simulink model "zrf_volt_4ant"  (R2019a)
settings: Solver=VariableStepAuto  StartTime=0.0  StopTime=10.0  RelTol=1e-3
libraries: xbsIndex_r4 x6321, casper_library_misc x95, xps_library x10, casper_library_delays x1
(part 1 of 63)
settings Model: Creator=jackh  LastModifiedBy=jackh

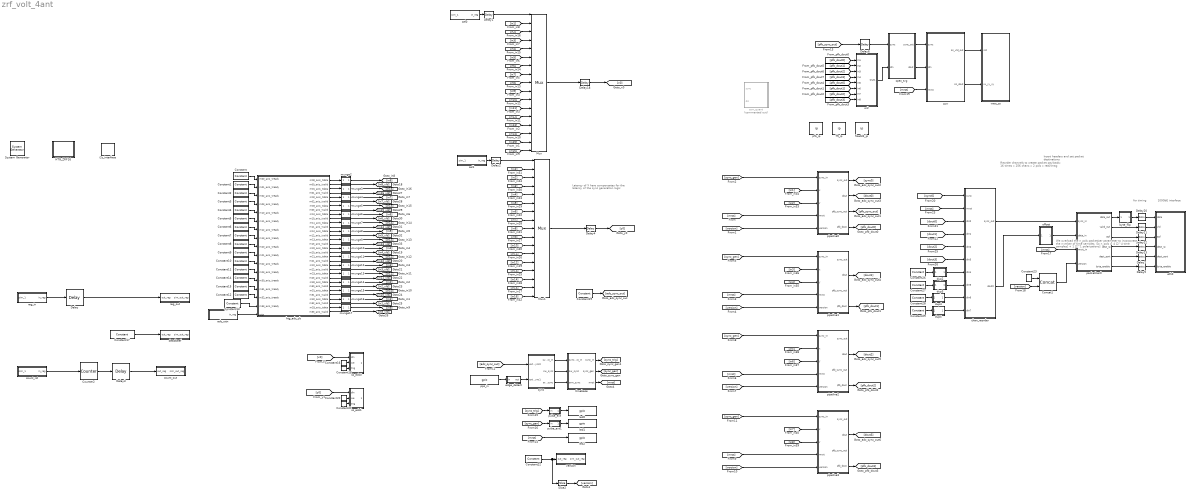
== system zrf_volt_4ant ==
  note: Latency of 5 here compensates
      | for the latency of the sync generation logic
  note: 100GbE interface
  note: for timing
  note: Insert headers and
      | set packet destinations
  note: We overload the n_pols packetizer
      | parameter to incorporate the number of time samples.
      | So n_pols = 4 [2^4 time samples] + 1 [2^1 polarizations]
  note: Reorder channels to
      | create packet payloads:
      | 16 times x 256 chans x 2 pols x real/imag
  " System Generator" : xbsIndex_r4/ System Generator  Tag=genX  xilinxfamily=zynquplusRFSOC  part=xczu49dr  speed=-2-e  package=ffvf1760  synthesis_tool=XST  clock_wrapper=Clock Enables  directory=/home/jackh/src/ata_rfsoc/zrf_volt_4ant/sysgen  proj_type=Vivado  Synth_file=Vivado Synthesis Defaults  Impl_file=Vivado Implementation Defaults  testbench=off  simulink_period=1  sysclk_period=3.9062  dcm_input_clock_period=10  incr_netlist=off  trim_vbits=Everywhere in SubSystem  dbl_ovrd=According to Block Masks  core_generation=According to Block Masks  run_coregen=off  deprecated_control=off  eval_field=0  block_type=sysgen
  Concat1 : xbsIndex_r4/Concat  num_inputs=2  dbl_ovrd=off  block_type=concat
  Constant{,1..15} (16 alike) : xbsIndex_r4/Constant  const=1  gui_display_data_type=Boolean  arith_type=Boolean  n_bits=1  bin_pt=0  preci_type=Single  exp_width=8  frac_width=24  explicit_period=on  period=1  equ=P=C  opselect=C  inp2=PCIN>>17  opr=+  inp1=P  carry=CIN  dbl_ovrd=off  block_type=constant
  Constant{16,18..21} (5 alike) : xbsIndex_r4/Constant  const=0  gui_display_data_type=Boolean  arith_type=Boolean  n_bits=16  bin_pt=14  preci_type=Single  exp_width=8  frac_width=24  explicit_period=on  period=1  equ=P=C  opselect=C  inp2=PCIN>>17  opr=+  inp1=P  carry=CIN  dbl_ovrd=off  block_type=constant
  Constant17 : xbsIndex_r4/Constant  const=hex2dec('deadbeef')  gui_display_data_type=Fixed-point  arith_type=Unsigned  n_bits=32  bin_pt=0  preci_type=Single  exp_width=8  frac_width=24  explicit_period=on  period=1  equ=P=C  opselect=C  inp2=PCIN>>17  opr=+  inp1=P  carry=CIN  dbl_ovrd=off  block_type=constant
  Constant22 : xbsIndex_r4/Constant  const=2  gui_display_data_type=Fixed-point  arith_type=Unsigned  n_bits=7  bin_pt=0  preci_type=Single  exp_width=8  frac_width=24  explicit_period=on  period=1  equ=P=C  opselect=C  inp2=PCIN>>17  opr=+  inp1=P  carry=CIN  dbl_ovrd=off  block_type=constant
  Constant23 : xbsIndex_r4/Constant  const=0  gui_display_data_type=Fixed-point  arith_type=Unsigned  n_bits=1  bin_pt=0  preci_type=Single  exp_width=8  frac_width=24  explicit_period=on  period=1  equ=P=C  opselect=C  inp2=PCIN>>17  opr=+  inp1=P  carry=CIN  dbl_ovrd=off  block_type=constant
  Constant26 : xbsIndex_r4/Constant  const=4  gui_display_data_type=Fixed-point  arith_type=Unsigned  n_bits=8  bin_pt=0  preci_type=Single  exp_width=8  frac_width=24  explicit_period=on  period=1  equ=P=C  opselect=C  inp2=PCIN>>17  opr=+  inp1=P  carry=CIN  dbl_ovrd=off  block_type=constant
  Constant27 : xbsIndex_r4/Constant  const=5  gui_display_data_type=Fixed-point  arith_type=Unsigned  n_bits=8  bin_pt=0  preci_type=Single  exp_width=8  frac_width=24  explicit_period=on  period=1  equ=P=C  opselect=C  inp2=PCIN>>17  opr=+  inp1=P  carry=CIN  dbl_ovrd=off  block_type=constant
  Constant28 : xbsIndex_r4/Constant  const=6  gui_display_data_type=Fixed-point  arith_type=Unsigned  n_bits=8  bin_pt=0  preci_type=Single  exp_width=8  frac_width=24  explicit_period=on  period=1  equ=P=C  opselect=C  inp2=PCIN>>17  opr=+  inp1=P  carry=CIN  dbl_ovrd=off  block_type=constant
  Constant29 : xbsIndex_r4/Constant  const=7  gui_display_data_type=Fixed-point  arith_type=Unsigned  n_bits=8  bin_pt=0  preci_type=Single  exp_width=8  frac_width=24  explicit_period=on  period=1  equ=P=C  opselect=C  inp2=PCIN>>17  opr=+  inp1=P  carry=CIN  dbl_ovrd=off  block_type=constant
  Counter2 : xbsIndex_r4/Counter  cnt_type=Free Running  cnt_to=Inf  operation=Up  start_count=0  cnt_by_val=1  arith_type=Unsigned  n_bits=32  bin_pt=0  load_pin=off  rst=on  en=off  explicit_period=on  period=1  use_behavioral_HDL=off  implementation=DSP48  dbl_ovrd=off  block_type=counter
  Delay{,1..3,5,7,20..23} (10 alike) : xbsIndex_r4/Delay  rst=off  infoeditControl=Selection of Reset will increase slice count due to use of real FFs and instead of SRLs  en=off  latency=1  reg_retiming=off  dbl_ovrd=off  block_type=delay
      Delay1 settings: block_version=11.4
      Delay2 settings: block_version=11.4
  Delay18 : xbsIndex_r4/Delay  rst=off  infoeditControl=Selection of Reset will increase slice count due to use of real FFs and instead of SRLs  en=off  latency=5  reg_retiming=off  dbl_ovrd=off  block_type=delay
      settings: block_version=11.4
  Delay4 : xbsIndex_r4/Delay  rst=off  infoeditControl=Selection of Reset will increase slice count due to use of real FFs and instead of SRLs  en=off  latency=5  reg_retiming=off  dbl_ovrd=off  block_type=delay
      settings: block_version=11.4
  Delay6 : xbsIndex_r4/Delay  rst=off  infoeditControl=Selection of Reset will increase slice count due to use of real FFs and instead of SRLs  en=off  latency=2  reg_retiming=off  dbl_ovrd=off  block_type=delay
  HTG_ZRF16 : Subsystem  Tag=xps:xsg  mask(xsg core config){hw_sys=htg_zrf16:xczu49dr, clk_src=adc_clk, clk_rate=256, sample_period=1, synthesis_tool=XST}
      mask prompts: hw_sys "Hardware Platform"; clk_src "User IP Clock source"; clk_rate "User IP Clock Rate (MHz)"; sample_period "Sample Period"; synthesis_tool "Synthesis Tool:"
      mask help:
      | The XSG Core Config block is used to configure the System Generator design
      | for the casper_xps toolflow. Settings here are used to configure the
      | Xilinx System Generator block parameters automatically, and control toolflow
      | script  execution. It needs to be at the top level of all designs being compiled
      | with the casper_xps toolflow.
      mask init:
      | xps_xsg_htg_zrf16_conf_mask;
      mask Help: eval('xlWeb([getenv(''MLIB_ROOT''), ''\doc\html\sys_xsg_core_config\sys_xsg_core_config.html''])')
      mask TypeOptions hw_sys: htg_zrf16:xczu29dr | htg_zrf16:xczu49dr
      mask TypeOptions clk_src: sys_clk | adc_clk | arb_clk
      mask TypeOptions synthesis_tool: Leonardo Spectrum | Synplify | Synplify Pro | XST
      mask Display: fprintf(['ZRF16']);
  Mux : xbsIndex_r4/Mux  inputs=16  en=off  latency=2  precision=Full  arith_type=Unsigned  n_bits=16  bin_pt=14  quantization=Truncate  overflow=Wrap  dbl_ovrd=off  block_type=mux
  Mux1 : xbsIndex_r4/Mux  inputs=16  en=off  latency=2  precision=Full  arith_type=Unsigned  n_bits=16  bin_pt=14  quantization=Truncate  overflow=Wrap  dbl_ovrd=off  block_type=mux
  Slice2 : xbsIndex_r4/Slice  nbits=7  boolean_output=off  mode=Lower Bit Location + Width  bit1=0  base1=MSB of Input  bit0=0  base0=LSB of Input  dbl_ovrd=off  block_type=slice
  adc_rstn : Subsystem  Tag=xps:sw_reg  AncestorBlock=xps_library/Memory/software_register  mask(swreg){io_dir=From Processor, io_delay=0, init_val=0, sample_period=1, names=reg, bitwidths=1, bin_pts=0, arith_types=2, sim_port=off, show_format=on}
      mask prompts: io_dir "I/O direction"; io_delay "I/O delay"; init_val "Initial Value"; sample_period "Sample period"; names "Bitfield names [msb...lsb]"; bitwidths "Bitfield widths"; bin_pts "Bitfield binary pts"; arith_types "Bitfield types, ufix=0, fix=1, bool=2"; sim_port "Provide sim input/output?"; show_format "Print format string?"
      mask help: A 32-bit software-accessible register. Can be divided into bitfields of varying widths and types using the fields in the block mask.
      mask init:
      | swreg_init(gcb)
      settings: AttributesFormatString=1input:b = 1 bits
      mask TypeOptions io_dir: To Processor | From Processor
      mask Callback io_dir:
      | mask_enables = get_param(gcb, 'MaskEnables');
      | mask_names = get_param(gcb, 'MaskNames');
      | if strcmp(get_param(gcb, 'io_dir'), 'To Processor'),
      |     mask_enables{ismember(mask_names, 'sample_period')} = 'off';
      | else
      |     mask_enables{ismember(mask_names, 'sample_period')} = 'on';
      | end
      | set_param(gcb, 'MaskEnables', mask_enables);
      mask DialogControl ParameterTabVar0 Prompt: Setup
  byte_flip : Subsystem  AncestorBlock=casper_library_flow_control/munge  mask(munge){divisions=64, div_size=8*ones(1,64), order=[63:-1:0], arith_type_out=Unsigned, bin_pt_out=0}
      mask prompts: divisions "Number of divisions"; div_size "Division size (bits)"; order "Division packing order"; arith_type_out "Output arithmetic type"; bin_pt_out "Output binary point"
      mask help: Splits an input bus into the specified number of divisions and then recombines them in the order specified (most significant division = 0,least = number divisions-1)
      mask init:
      | munge_init(gcb, ...
      |     'divisions', divisions, ...
      |     'div_size', div_size, ...
      |     'order', order, ...
      |     'arith_type_out', arith_type_out, ...
      |     'bin_pt_out', bin_pt_out);
      settings: AttributesFormatString=|
      | split:[8 8 8 8 8 8 8 8 8 8 8 8 8 8 8 8 8 8 8 8 8 8 8 8 8 8 8 8 8 8 8 8 8 8 8 8 8 8 8 8 8 8 8 8 8 8 8 8 8 8 8 8 8 8 8 8 8 8 8 8 8 8 8 8]
      | join:[63 62 61 60 59 58 57 56 55 54 53 52 51 50 49 48 47 46 45 44 43 42 41 40 39 38 37 36 35 34 33 32 31 30 29 28 27 26 25 24 23 22 21 20 19 18 17 16 15 14 13 12 11 10 9 8 7 6 5 4 3 2 1 0]
      | Unsigned [512,0]
      mask TypeOptions arith_type_out: Unsigned | Signed  (2's comp) | Floating-point
  chan_reorder : Subsystem
  corr : Subsystem  mask{n_chan_bits=12}
      mask prompts: n_chan_bits "Number of channels? (2^?)"
  corr_quant : Subsystem  Commented=on  mask{n_chan_bits=12}
      mask prompts: n_chan_bits "Number of channels? (2^?)"
  count_out : Subsystem  Tag=xps:sw_reg  AncestorBlock=xps_library/Memory/software_register  mask(swreg){io_dir=To Processor, io_delay=0, init_val=0, sample_period=1, names=reg, bitwidths=32, bin_pts=0, arith_types=0, sim_port=on, show_format=on}
      mask prompts: io_dir "I/O direction"; io_delay "I/O delay"; init_val "Initial Value"; sample_period "Sample period"; names "Bitfield names [msb...lsb]"; bitwidths "Bitfield widths"; bin_pts "Bitfield binary pts"; arith_types "Bitfield types, ufix=0, fix=1, bool=2"; sim_port "Provide sim input/output?"; show_format "Print format string?"
      mask help: A 32-bit software-accessible register. Can be divided into bitfields of varying widths and types using the fields in the block mask.
      mask init:
      | swreg_init(gcb)
      settings: AttributesFormatString=1output:uf32.0 = 32 bits
      mask TypeOptions io_dir: To Processor | From Processor
      mask Callback io_dir:
      | mask_enables = get_param(gcb, 'MaskEnables');
      | mask_names = get_param(gcb, 'MaskNames');
      | if strcmp(get_param(gcb, 'io_dir'), 'To Processor'),
      |     mask_enables{ismember(mask_names, 'sample_period')} = 'off';
      | else
      |     mask_enables{ismember(mask_names, 'sample_period')} = 'on';
      | end
      | set_param(gcb, 'MaskEnables', mask_enables);
      mask DialogControl ParameterTabVar0 Prompt: Setup
  count_rst : Subsystem  Tag=xps:sw_reg  AncestorBlock=xps_library/Memory/software_register  mask(swreg){io_dir=From Processor, io_delay=0, init_val=0, sample_period=1, names=reg, bitwidths=1, bin_pts=0, arith_types=2, sim_port=on, show_format=on}
      mask prompts: io_dir "I/O direction"; io_delay "I/O delay"; init_val "Initial Value"; sample_period "Sample period"; names "Bitfield names [msb...lsb]"; bitwidths "Bitfield widths"; bin_pts "Bitfield binary pts"; arith_types "Bitfield types, ufix=0, fix=1, bool=2"; sim_port "Provide sim input/output?"; show_format "Print format string?"
      mask help: A 32-bit software-accessible register. Can be divided into bitfields of varying widths and types using the fields in the block mask.
      mask init:
      | swreg_init(gcb)
      settings: AttributesFormatString=1input:b = 1 bits
      mask TypeOptions io_dir: To Processor | From Processor
      mask Callback io_dir:
      | mask_enables = get_param(gcb, 'MaskEnables');
      | mask_names = get_param(gcb, 'MaskNames');
      | if strcmp(get_param(gcb, 'io_dir'), 'To Processor'),
      |     mask_enables{ismember(mask_names, 'sample_period')} = 'off';
      | else
      |     mask_enables{ismember(mask_names, 'sample_period')} = 'on';
      | end
      | set_param(gcb, 'MaskEnables', mask_enables);
      mask DialogControl ParameterTabVar0 Prompt: Setup
  deadbeef : Subsystem  Tag=xps:sw_reg  AncestorBlock=xps_library/Memory/software_register  mask(swreg){io_dir=To Processor, io_delay=0, init_val=0, sample_period=1, names=reg, bitwidths=32, bin_pts=0, arith_types=0, sim_port=on, show_format=on}
      mask prompts: io_dir "I/O direction"; io_delay "I/O delay"; init_val "Initial Value"; sample_period "Sample period"; names "Bitfield names [msb...lsb]"; bitwidths "Bitfield widths"; bin_pts "Bitfield binary pts"; arith_types "Bitfield types, ufix=0, fix=1, bool=2"; sim_port "Provide sim input/output?"; show_format "Print format string?"
      mask help: A 32-bit software-accessible register. Can be divided into bitfields of varying widths and types using the fields in the block mask.
      mask init:
      | swreg_init(gcb)
      settings: AttributesFormatString=1output:uf32.0 = 32 bits
      mask TypeOptions io_dir: To Processor | From Processor
      mask Callback io_dir:
      | mask_enables = get_param(gcb, 'MaskEnables');
      | mask_names = get_param(gcb, 'MaskNames');
      | if strcmp(get_param(gcb, 'io_dir'), 'To Processor'),
      |     mask_enables{ismember(mask_names, 'sample_period')} = 'off';
      | else
      |     mask_enables{ismember(mask_names, 'sample_period')} = 'on';
      | end
      | set_param(gcb, 'MaskEnables', mask_enables);
      mask DialogControl ParameterTabVar0 Prompt: Setup
  dup2 : Subsystem
  dup3 : Subsystem
  dup4 : Subsystem
  dup5 : Subsystem
  edge_detect : Subsystem  AncestorBlock=casper_library_misc/edge_detect  mask(edge_detect){edge=Rising, polarity=Active High, x_in=[0 0.08 0.08 0.16 0.16 0.24 0.24 0.32 0.32 0.4], y_in=[-1 -1  1  1  1  1  1  1  1  1], x_out=[0.6 0.68 0.68 0.76 0.76 0.84 0.84 0.92 0.92 1], y_out=[-1 -1  1  1 -1 -1 -1 -1 -1 -1]}
      mask prompts: edge "Edge Type"; polarity "Output Polarity"; x_in "Input X Positions"; y_in "Input Y Positions"; x_out "Output X Positions"; y_out "Output Y Positions"
      mask help: Output is active for one-cycle after each edge of the specified type (i.e. rising, falling or both).
      mask init:
      | edge_detect_init(gcb,...
      |     'edge',edge,...
      |     'polarity',polarity,...
      |     'x_in',x_in,...
      |     'x_out',x_out,...
      |     'y_in',y_in,...
      |     'y_out',y_out);
      | 
      | x_in_num=str2num(getfield(getfield(get_param(gcb,'UserData'),'parameters'),'x_in'));
      | x_out_num=str2num(getfield(getfield(get_param(gcb,'UserData'),'parameters'),'x_out'));
      | y_in_num=str2num(getfield(getfield(get_param(gcb,'UserData'),'parameters'),'y_in'));
      | y_out_num=str2num(getfield(getfield(get_param(gcb,'UserData'),'parameters'),'y_out'));
      settings: AttributesFormatString=|
      | rising edges
      | active high
      mask Help: Output is active for one-cycle after each edge of the specified type (i.e. rising, falling, or both).  Latency is zero.
      mask TypeOptions edge: Rising | Falling | Both
      mask TypeOptions polarity: Active High | Active Low
      mask Display:
      | plot(x_in_num,0.5+y_in_num*0.2);
      | plot(x_out_num,0.5+y_out_num*0.2);
  eth0 : Subsystem
  fft_ip : xps_library/Utilities/ip  Tag=xps:ip  lib_path=[fileparts(which(bdroot)) '/fft_4096c_2i_core']  ip_name='fft_4096c_2i_core'
      settings: SourceProductName=CASPER XPS Blockset
  float32_ip : xps_library/Utilities/ip  Tag=xps:ip  lib_path=[fileparts(which(bdroot)) '/int64_to_float32_latency6_core']  ip_name='int64_to_float32_latency6_core'
      settings: SourceProductName=CASPER XPS Blockset
  htg_adc_yb : Subsystem  Tag=xps:adc_htgzrf16  mask(htg_adc){tile_224_enable_pll=on, tile_224_sample_rate=4096, tile_224_clk_out=256.000, tile_224_ref_clk=512.000, tile_224_axi_stream_clk=0, tile_224_adc_0=on, tile_224_adc0_digital_output=I/Q, tile_224_adc0_dec_mode=2x, tile_224_adc0_sample_per_cycle=8, tile_224_adc0_req_axis_clk=0, tile_224_adc_1=on, tile_224_adc1_digital_output=I/Q, tile_224_adc1_dec_mode=2x, tile_224_adc1_sample_per_cycle=8, tile_224_adc1_req_axis_clk=0, tile_225_enable_pll=on, tile_225_sample_rate=4096, tile_225_clk_out=256.000, tile_225_ref_clk=512.000, tile_225_axi_stream_clk=0, tile_225_adc_0=on, tile_225_adc0_digital_output=I/Q, tile_225_adc0_dec_mode=2x, tile_225_adc0_sample_per_cycle=8, tile_225_adc0_req_axis_clk=0, tile_225_adc_1=on, tile_225_adc1_digital_output=I/Q, tile_225_adc1_dec_mode=2x, tile_225_adc1_sample_per_cycle=8, tile_225_adc1_req_axis_clk=0, tile_226_enable_pll=on, tile_226_sample_rate=4096, tile_226_clk_out=256.000, tile_226_ref_clk=512.000, tile_226_axi_stream_clk=0, tile_226_adc_0=on, tile_226_adc0_digital_output=I/Q, tile_226_adc0_dec_mode=2x, tile_226_adc0_sample_per_cycle=8, tile_226_adc0_req_axis_clk=0, tile_226_adc_1=on, tile_226_adc1_digital_output=I/Q, tile_226_adc1_dec_mode=2x, tile_226_adc1_sample_per_cycle=8, tile_226_adc1_req_axis_clk=0, tile_227_enable_pll=on, tile_227_sample_rate=4096, tile_227_clk_out=256.000, tile_227_ref_clk=512.000, tile_227_axi_stream_clk=0, tile_227_adc_0=on, tile_227_adc0_digital_output=I/Q, tile_227_adc0_dec_mode=2x, tile_227_adc0_sample_per_cycle=8, tile_227_adc0_req_axis_clk=0, tile_227_adc_1=on, tile_227_adc1_digital_output=I/Q, tile_227_adc1_dec_mode=2x, tile_227_adc1_sample_per_cycle=8, tile_227_adc1_req_axis_clk=0}
      mask prompts: tile_224_enable_pll "Enable PLL"; tile_224_sample_rate "Sampling Rate (MSPS)"; tile_224_clk_out "Clock Out (MHz)"; tile_224_ref_clk "Reference Clock (MHz)"; tile_224_axi_stream_clk "AXI4-Stream Clock (MHz)"; tile_224_adc_0 "Enable ADC"; tile_224_adc0_digital_output "Digital Output Data"; tile_224_adc0_dec_mode "Decimation Mode"; tile_224_adc0_sample_per_cycle "Samples per AXI4-Stream Cycle"; tile_224_adc_1 "Enable ADC"; tile_224_adc1_digital_output "Digital Output Data"; tile_224_adc1_dec_mode "Decimation Mode"; tile_224_adc1_sample_per_cycle "Samples per AXI4-Stream Cycle"; tile_225_enable_pll "Enable PLL"; tile_225_sample_rate "Sampling Rate (MSPS)"; tile_225_clk_out "Clock Out (MHz)"; tile_225_ref_clk "Reference Clock (MHz)"; tile_225_axi_stream_clk "AXI4-Stream Clock (MHz)"; tile_225_adc_0 "Enable ADC"; tile_225_adc0_digital_output "Digital Output Data"; tile_225_adc0_dec_mode "Decimation Mode"; tile_225_adc0_sample_per_cycle "Samples per AXI4-Stream Cycle"; tile_225_adc_1 "Enable ADC"; tile_225_adc1_digital_output "Digital Output Data"; tile_225_adc1_dec_mode "Decimation Mode"; tile_225_adc1_sample_per_cycle "Samples per AXI4-Stream Cycle"; tile_226_enable_pll "Enable PLL"; tile_226_sample_rate "Sampling Rate (MSPS)"; tile_226_clk_out "Clock Out (MHz)"; tile_226_ref_clk "Reference Clock (MHz)"; tile_226_axi_stream_clk "AXI4-Stream Clock (MHz)"; tile_226_adc_0 "Enable ADC"; tile_226_adc0_digital_output "Digital Output Data"; tile_226_adc0_dec_mode "Decimation Mode"; tile_226_adc0_sample_per_cycle "Samples per AXI4-Stream Cycle"; tile_226_adc_1 "Enable ADC"; tile_226_adc1_digital_output "Digital Output Data"; tile_226_adc1_dec_mode "Decimation Mode"; tile_226_adc1_sample_per_cycle "Samples per AXI4-Stream Cycle"; tile_227_enable_pll "Enable PLL"; tile_227_sample_rate "Sampling Rate (MSPS)"; tile_227_clk_out "Clock Out (MHz)"; tile_227_ref_clk "Reference Clock (MHz)"; tile_227_axi_stream_clk "AXI4-Stream Clock (MHz)"; tile_227_adc_0 "Enable ADC"; tile_227_adc0_digital_output "Digital Output Data"; tile_227_adc0_dec_mode "Decimation Mode"; tile_227_adc0_sample_per_cycle "Samples per AXI4-Stream Cycle"; tile_227_adc_1 "Enable ADC"; tile_227_adc1_digital_output "Digital Output Data"; tile_227_adc1_dec_mode "Decimation Mode"; tile_227_adc1_sample_per_cycle "Samples per AXI4-Stream Cycle"
      mask init:
      | htg_adc_mask(gcb)
      mask Help: eval('xlWeb([getenv(''MLIB_ROOT''), ''\doc\html\adc_zcu111\adc_zcu111.html''])')
      mask TypeOptions tile_224_clk_out: 32.000 | 64.000 | 128.000 | 256.000
      mask TypeOptions tile_224_ref_clk: 103.261 | 104.136 | 105.026 | 105.931 | 106.852 | 107.790 | 108.743 | 109.714 | 110.703 | 111.709 | 112.734 | 113.778 | 114.841 | 115.925 | 117.029 | 118.154 | 119.301 | 120.471 | 121.663 | 122.880 | 124.121 | 125.388 | 126.680 | 128.000 | 129.347 | 130.723 | 132.129 | 133.565 | 135.033 | 136.533 | 138.067 | 139.636 | 141.241 | 142.884 | 144.565 | 146.286 | 148.048 | 149.854 | 151.704 | 153.600 | 155.544 | 157.539 | 159.584 | 161.684 | 163.840 | 166.054 | 168.329 | 170.667 | 173.070 | 175.543 | 178.087 | 180.706 | 183.403 | 186.182 | 189.046 | 192.000 | 195.048 | 198.194 | 201.443 | 204.800 | 208.271 | 211.862 | 215.579 | 219.429 | 223.418 | 227.556 | 231.849 | 236.308 | 240.941 | 245.760 | 250.776 | 256.000 | 261.447 | 267.130 | 273.067 | 279.273 | 285.767 | 292.571 | 299.707 | 307.200 | 315.077 | 323.368 | 332.108 | 341.333 | 351.086 | 361.412 | 372.364 | 384.000 | 396.387 | 409.600 | 423.724 | 438.857 | 455.111 | 472.615 | 491.520 | 512.000 | 534.261 | 558.546 | 585.143 | 614.400 | 646.737 | 682.667 | 722.824 | 768.000
      mask TypeOptions tile_224_adc0_digital_output: I/Q | Real
      mask TypeOptions tile_224_adc0_dec_mode: 1x | 2x | 4x | 8x
      mask TypeOptions tile_224_adc0_sample_per_cycle: 1 | 2 | 3 | 4 | 5 | 6 | 7 | 8
      mask TypeOptions tile_224_adc1_digital_output: I/Q | Real
      mask TypeOptions tile_224_adc1_dec_mode: 1x | 2x | 4x | 8x
      mask TypeOptions tile_224_adc1_sample_per_cycle: 1 | 2 | 3 | 4 | 5 | 6 | 7 | 8
      mask TypeOptions tile_225_clk_out: 32.000 | 64.000 | 128.000 | 256.000
      mask TypeOptions tile_225_ref_clk: 103.261 | 104.136 | 105.026 | 105.931 | 106.852 | 107.790 | 108.743 | 109.714 | 110.703 | 111.709 | 112.734 | 113.778 | 114.841 | 115.925 | 117.029 | 118.154 | 119.301 | 120.471 | 121.663 | 122.880 | 124.121 | 125.388 | 126.680 | 128.000 | 129.347 | 130.723 | 132.129 | 133.565 | 135.033 | 136.533 | 138.067 | 139.636 | 141.241 | 142.884 | 144.565 | 146.286 | 148.048 | 149.854 | 151.704 | 153.600 | 155.544 | 157.539 | 159.584 | 161.684 | 163.840 | 166.054 | 168.329 | 170.667 | 173.070 | 175.543 | 178.087 | 180.706 | 183.403 | 186.182 | 189.046 | 192.000 | 195.048 | 198.194 | 201.443 | 204.800 | 208.271 | 211.862 | 215.579 | 219.429 | 223.418 | 227.556 | 231.849 | 236.308 | 240.941 | 245.760 | 250.776 | 256.000 | 261.447 | 267.130 | 273.067 | 279.273 | 285.767 | 292.571 | 299.707 | 307.200 | 315.077 | 323.368 | 332.108 | 341.333 | 351.086 | 361.412 | 372.364 | 384.000 | 396.387 | 409.600 | 423.724 | 438.857 | 455.111 | 472.615 | 491.520 | 512.000 | 534.261 | 558.546 | 585.143 | 614.400 | 646.737 | 682.667 | 722.824 | 768.000
      mask TypeOptions tile_225_adc0_digital_output: I/Q | Real
      mask TypeOptions tile_225_adc0_dec_mode: 1x | 2x | 4x | 8x
      mask TypeOptions tile_225_adc0_sample_per_cycle: 1 | 2 | 3 | 4 | 5 | 6 | 7 | 8
      mask TypeOptions tile_225_adc1_digital_output: I/Q | Real
      mask TypeOptions tile_225_adc1_dec_mode: 1x | 2x | 4x | 8x
      mask TypeOptions tile_225_adc1_sample_per_cycle: 1 | 2 | 3 | 4 | 5 | 6 | 7 | 8
      mask TypeOptions tile_226_clk_out: 32.000 | 64.000 | 128.000 | 256.000
      mask TypeOptions tile_226_ref_clk: 103.261 | 104.136 | 105.026 | 105.931 | 106.852 | 107.790 | 108.743 | 109.714 | 110.703 | 111.709 | 112.734 | 113.778 | 114.841 | 115.925 | 117.029 | 118.154 | 119.301 | 120.471 | 121.663 | 122.880 | 124.121 | 125.388 | 126.680 | 128.000 | 129.347 | 130.723 | 132.129 | 133.565 | 135.033 | 136.533 | 138.067 | 139.636 | 141.241 | 142.884 | 144.565 | 146.286 | 148.048 | 149.854 | 151.704 | 153.600 | 155.544 | 157.539 | 159.584 | 161.684 | 163.840 | 166.054 | 168.329 | 170.667 | 173.070 | 175.543 | 178.087 | 180.706 | 183.403 | 186.182 | 189.046 | 192.000 | 195.048 | 198.194 | 201.443 | 204.800 | 208.271 | 211.862 | 215.579 | 219.429 | 223.418 | 227.556 | 231.849 | 236.308 | 240.941 | 245.760 | 250.776 | 256.000 | 261.447 | 267.130 | 273.067 | 279.273 | 285.767 | 292.571 | 299.707 | 307.200 | 315.077 | 323.368 | 332.108 | 341.333 | 351.086 | 361.412 | 372.364 | 384.000 | 396.387 | 409.600 | 423.724 | 438.857 | 455.111 | 472.615 | 491.520 | 512.000 | 534.261 | 558.546 | 585.143 | 614.400 | 646.737 | 682.667 | 722.824 | 768.000
      mask TypeOptions tile_226_adc0_digital_output: I/Q | Real
      mask TypeOptions tile_226_adc0_dec_mode: 1x | 2x | 4x | 8x
      mask TypeOptions tile_226_adc0_sample_per_cycle: 1 | 2 | 3 | 4 | 5 | 6 | 7 | 8
      mask TypeOptions tile_226_adc1_digital_output: I/Q | Real
      mask TypeOptions tile_226_adc1_dec_mode: 1x | 2x | 4x | 8x
      mask TypeOptions tile_226_adc1_sample_per_cycle: 1 | 2 | 3 | 4 | 5 | 6 | 7 | 8
      mask TypeOptions tile_227_clk_out: 32.000 | 64.000 | 128.000 | 256.000
      mask TypeOptions tile_227_ref_clk: 103.261 | 104.136 | 105.026 | 105.931 | 106.852 | 107.790 | 108.743 | 109.714 | 110.703 | 111.709 | 112.734 | 113.778 | 114.841 | 115.925 | 117.029 | 118.154 | 119.301 | 120.471 | 121.663 | 122.880 | 124.121 | 125.388 | 126.680 | 128.000 | 129.347 | 130.723 | 132.129 | 133.565 | 135.033 | 136.533 | 138.067 | 139.636 | 141.241 | 142.884 | 144.565 | 146.286 | 148.048 | 149.854 | 151.704 | 153.600 | 155.544 | 157.539 | 159.584 | 161.684 | 163.840 | 166.054 | 168.329 | 170.667 | 173.070 | 175.543 | 178.087 | 180.706 | 183.403 | 186.182 | 189.046 | 192.000 | 195.048 | 198.194 | 201.443 | 204.800 | 208.271 | 211.862 | 215.579 | 219.429 | 223.418 | 227.556 | 231.849 | 236.308 | 240.941 | 245.760 | 250.776 | 256.000 | 261.447 | 267.130 | 273.067 | 279.273 | 285.767 | 292.571 | 299.707 | 307.200 | 315.077 | 323.368 | 332.108 | 341.333 | 351.086 | 361.412 | 372.364 | 384.000 | 396.387 | 409.600 | 423.724 | 438.857 | 455.111 | 472.615 | 491.520 | 512.000 | 534.261 | 558.546 | 585.143 | 614.400 | 646.737 | 682.667 | 722.824 | 768.000
      mask TypeOptions tile_227_adc0_digital_output: I/Q | Real
      mask TypeOptions tile_227_adc0_dec_mode: 1x | 2x | 4x | 8x
      mask TypeOptions tile_227_adc0_sample_per_cycle: 1 | 2 | 3 | 4 | 5 | 6 | 7 | 8
      mask TypeOptions tile_227_adc1_digital_output: I/Q | Real
      mask TypeOptions tile_227_adc1_dec_mode: 1x | 2x | 4x | 8x
      mask TypeOptions tile_227_adc1_sample_per_cycle: 1 | 2 | 3 | 4 | 5 | 6 | 7 | 8
      mask DialogControl adc_tile_224 Prompt: ADC Tile 224
      mask DialogControl pll_clocking_config_224 Prompt: PLL and Clocking Configuration
      mask DialogControl tile_224_adc0 Prompt: ADC 0
      mask DialogControl tile_224_adc0_data_settings Prompt: Data Settings
      mask DialogControl tile_224_adc0_req_axis_clk_label Prompt: Required AXI4-Stream clock:
      mask DialogControl tile_224_adc1 Prompt: ADC 1
      mask DialogControl tile_224_adc1_data_settings Prompt: Data Settings
      mask DialogControl tile_224_adc1_req_axis_clk_label Prompt: Required AXI4-Stream clock:
      mask DialogControl adc_tile_225 Prompt: ADC Tile 225
      mask DialogControl pll_clocking_config_225 Prompt: PLL and Clocking Configuration
      mask DialogControl tile_225_adc0 Prompt: ADC 0
      mask DialogControl tile_225_adc0_data_settings Prompt: Data Settings
      mask DialogControl tile_225_adc0_req_axis_clk_label Prompt: Required AXI4-Stream clock:
      mask DialogControl tile_225_adc1 Prompt: ADC 1
      mask DialogControl tile_225_adc1_data_settings Prompt: Data Settings
      mask DialogControl tile_225_adc1_req_axis_clk_label Prompt: Required AXI4-Stream clock:
      mask DialogControl adc_tile_226 Prompt: ADC Tile 226
      mask DialogControl pll_clocking_config_226 Prompt: PLL and Clocking Configuration
      mask DialogControl tile_226_adc0 Prompt: ADC 0
      mask DialogControl tile_226_adc0_data_settings Prompt: Data Settings
      mask DialogControl tile_226_adc0_req_axis_clk_label Prompt: Required AXI4-Stream clock:
      mask DialogControl tile_226_adc1 Prompt: ADC 1
      mask DialogControl tile_226_adc1_data_settings Prompt: Data Settings
      mask DialogControl tile_226_adc1_req_axis_clk_label Prompt: Required AXI4-Stream clock:
      mask DialogControl adc_tile_227 Prompt: ADC Tile 227
      mask DialogControl pll_clocking_config_227 Prompt: PLL and Clocking Configuration
      mask DialogControl tile_227_adc0 Prompt: ADC 0
      mask DialogControl tile_227_adc0_data_settings Prompt: Data Settings
      mask DialogControl tile_227_adc0_req_axis_clk_label Prompt: Required AXI4-Stream clock:
      mask DialogControl tile_227_adc1 Prompt: ADC 1
      mask DialogControl tile_227_adc1_data_settings Prompt: Data Settings
      mask DialogControl tile_227_adc1_req_axis_clk_label Prompt: Required AXI4-Stream clock:
  i2c_interface : xps_library/IO/i2c_interface  Tag=xps:i2c_interface  sda_gpio='i2c'  sda_gpio_index=0  scl_gpio='i2c'  scl_gpio_index=1
      settings: SourceProductName=CASPER XPS Blockset
  led0 : xps_library/IO/gpio  Tag=xps:gpio  io_group_params_forwarded=on  io_group=ROACH:led  io_group_real=led  io_group_custom=0  io_dir=out  arith_type=Boolean  bitwidth=1  bin_pt=0  bit_index=0  sample_period=1  use_single_ended=off  use_ddr=off  reg_iob=on  reg_clk_phase=0  termination=None
      settings: SourceProductName=CASPER XPS Blockset
  led1 : xps_library/IO/gpio  Tag=xps:gpio  io_group_params_forwarded=on  io_group=ROACH:led  io_group_real=led  io_group_custom=0  io_dir=out  arith_type=Boolean  bitwidth=1  bin_pt=0  bit_index=1  sample_period=1  use_single_ended=off  use_ddr=off  reg_iob=on  reg_clk_phase=0  termination=None
      settings: SourceProductName=CASPER XPS Blockset
  led2 : xps_library/IO/gpio  Tag=xps:gpio  io_group_params_forwarded=on  io_group=ROACH:led  io_group_real=led  io_group_custom=0  io_dir=out  arith_type=Boolean  bitwidth=1  bin_pt=0  bit_index=2  sample_period=1  use_single_ended=off  use_ddr=off  reg_iob=on  reg_clk_phase=0  termination=None
      settings: SourceProductName=CASPER XPS Blockset
  munge10 : Subsystem  AncestorBlock=casper_library_flow_control/munge  mask(munge){divisions=8, div_size=[16 16 16 16 16 16 16 16], order=[7 6 5 4 3 2 1 0], arith_type_out=Unsigned, bin_pt_out=0}
      mask prompts: divisions "Number of divisions"; div_size "Division size (bits)"; order "Division packing order"; arith_type_out "Output arithmetic type"; bin_pt_out "Output binary point"
      mask help: Splits an input bus into the specified number of divisions and then recombines them in the order specified (most significant division = 0,least = number divisions-1)
      mask init:
      | munge_init(gcb, ...
      |     'divisions', divisions, ...
      |     'div_size', div_size, ...
      |     'order', order, ...
      |     'arith_type_out', arith_type_out, ...
      |     'bin_pt_out', bin_pt_out);
      settings: AttributesFormatString=|
      | split:[16 16 16 16 16 16 16 16]
      | join:[7 6 5 4 3 2 1 0]
      | Unsigned [128,0]
      mask TypeOptions arith_type_out: Unsigned | Signed  (2's comp) | Floating-point
  munge11 : Subsystem  AncestorBlock=casper_library_flow_control/munge  mask(munge){divisions=8, div_size=[16 16 16 16 16 16 16 16], order=[7 6 5 4 3 2 1 0], arith_type_out=Unsigned, bin_pt_out=0}
      mask prompts: divisions "Number of divisions"; div_size "Division size (bits)"; order "Division packing order"; arith_type_out "Output arithmetic type"; bin_pt_out "Output binary point"
      mask help: Splits an input bus into the specified number of divisions and then recombines them in the order specified (most significant division = 0,least = number divisions-1)
      mask init:
      | munge_init(gcb, ...
      |     'divisions', divisions, ...
      |     'div_size', div_size, ...
      |     'order', order, ...
      |     'arith_type_out', arith_type_out, ...
      |     'bin_pt_out', bin_pt_out);
      settings: AttributesFormatString=|
      | split:[16 16 16 16 16 16 16 16]
      | join:[7 6 5 4 3 2 1 0]
      | Unsigned [128,0]
      mask TypeOptions arith_type_out: Unsigned | Signed  (2's comp) | Floating-point
  munge12 : Subsystem  AncestorBlock=casper_library_flow_control/munge  mask(munge){divisions=8, div_size=[16 16 16 16 16 16 16 16], order=[7 6 5 4 3 2 1 0], arith_type_out=Unsigned, bin_pt_out=0}
      mask prompts: divisions "Number of divisions"; div_size "Division size (bits)"; order "Division packing order"; arith_type_out "Output arithmetic type"; bin_pt_out "Output binary point"
      mask help: Splits an input bus into the specified number of divisions and then recombines them in the order specified (most significant division = 0,least = number divisions-1)
      mask init:
      | munge_init(gcb, ...
      |     'divisions', divisions, ...
      |     'div_size', div_size, ...
      |     'order', order, ...
      |     'arith_type_out', arith_type_out, ...
      |     'bin_pt_out', bin_pt_out);
      settings: AttributesFormatString=|
      | split:[16 16 16 16 16 16 16 16]
      | join:[7 6 5 4 3 2 1 0]
      | Unsigned [128,0]
      mask TypeOptions arith_type_out: Unsigned | Signed  (2's comp) | Floating-point
  munge13 : Subsystem  AncestorBlock=casper_library_flow_control/munge  mask(munge){divisions=8, div_size=[16 16 16 16 16 16 16 16], order=[7 6 5 4 3 2 1 0], arith_type_out=Unsigned, bin_pt_out=0}
      mask prompts: divisions "Number of divisions"; div_size "Division size (bits)"; order "Division packing order"; arith_type_out "Output arithmetic type"; bin_pt_out "Output binary point"
      mask help: Splits an input bus into the specified number of divisions and then recombines them in the order specified (most significant division = 0,least = number divisions-1)
      mask init:
      | munge_init(gcb, ...
      |     'divisions', divisions, ...
      |     'div_size', div_size, ...
      |     'order', order, ...
      |     'arith_type_out', arith_type_out, ...
      |     'bin_pt_out', bin_pt_out);
      settings: AttributesFormatString=|
      | split:[16 16 16 16 16 16 16 16]
      | join:[7 6 5 4 3 2 1 0]
      | Unsigned [128,0]
      mask TypeOptions arith_type_out: Unsigned | Signed  (2's comp) | Floating-point
  munge14 : Subsystem  AncestorBlock=casper_library_flow_control/munge  mask(munge){divisions=8, div_size=[16 16 16 16 16 16 16 16], order=[7 6 5 4 3 2 1 0], arith_type_out=Unsigned, bin_pt_out=0}
      mask prompts: divisions "Number of divisions"; div_size "Division size (bits)"; order "Division packing order"; arith_type_out "Output arithmetic type"; bin_pt_out "Output binary point"
      mask help: Splits an input bus into the specified number of divisions and then recombines them in the order specified (most significant division = 0,least = number divisions-1)
      mask init:
      | munge_init(gcb, ...
      |     'divisions', divisions, ...
      |     'div_size', div_size, ...
      |     'order', order, ...
      |     'arith_type_out', arith_type_out, ...
      |     'bin_pt_out', bin_pt_out);
      settings: AttributesFormatString=|
      | split:[16 16 16 16 16 16 16 16]
      | join:[7 6 5 4 3 2 1 0]
      | Unsigned [128,0]
      mask TypeOptions arith_type_out: Unsigned | Signed  (2's comp) | Floating-point
  munge15 : Subsystem  AncestorBlock=casper_library_flow_control/munge  mask(munge){divisions=8, div_size=[16 16 16 16 16 16 16 16], order=[7 6 5 4 3 2 1 0], arith_type_out=Unsigned, bin_pt_out=0}
      mask prompts: divisions "Number of divisions"; div_size "Division size (bits)"; order "Division packing order"; arith_type_out "Output arithmetic type"; bin_pt_out "Output binary point"
      mask help: Splits an input bus into the specified number of divisions and then recombines them in the order specified (most significant division = 0,least = number divisions-1)
      mask init:
      | munge_init(gcb, ...
      |     'divisions', divisions, ...
      |     'div_size', div_size, ...
      |     'order', order, ...
      |     'arith_type_out', arith_type_out, ...
      |     'bin_pt_out', bin_pt_out);
      settings: AttributesFormatString=|
      | split:[16 16 16 16 16 16 16 16]
      | join:[7 6 5 4 3 2 1 0]
      | Unsigned [128,0]
      mask TypeOptions arith_type_out: Unsigned | Signed  (2's comp) | Floating-point
  munge16 : Subsystem  AncestorBlock=casper_library_flow_control/munge  mask(munge){divisions=8, div_size=[16 16 16 16 16 16 16 16], order=[7 6 5 4 3 2 1 0], arith_type_out=Unsigned, bin_pt_out=0}
      mask prompts: divisions "Number of divisions"; div_size "Division size (bits)"; order "Division packing order"; arith_type_out "Output arithmetic type"; bin_pt_out "Output binary point"
      mask help: Splits an input bus into the specified number of divisions and then recombines them in the order specified (most significant division = 0,least = number divisions-1)
      mask init:
      | munge_init(gcb, ...
      |     'divisions', divisions, ...
      |     'div_size', div_size, ...
      |     'order', order, ...
      |     'arith_type_out', arith_type_out, ...
      |     'bin_pt_out', bin_pt_out);
      settings: AttributesFormatString=|
      | split:[16 16 16 16 16 16 16 16]
      | join:[7 6 5 4 3 2 1 0]
      | Unsigned [128,0]
      mask TypeOptions arith_type_out: Unsigned | Signed  (2's comp) | Floating-point
  munge17 : Subsystem  AncestorBlock=casper_library_flow_control/munge  mask(munge){divisions=8, div_size=[16 16 16 16 16 16 16 16], order=[7 6 5 4 3 2 1 0], arith_type_out=Unsigned, bin_pt_out=0}
      mask prompts: divisions "Number of divisions"; div_size "Division size (bits)"; order "Division packing order"; arith_type_out "Output arithmetic type"; bin_pt_out "Output binary point"
      mask help: Splits an input bus into the specified number of divisions and then recombines them in the order specified (most significant division = 0,least = number divisions-1)
      mask init:
      | munge_init(gcb, ...
      |     'divisions', divisions, ...
      |     'div_size', div_size, ...
      |     'order', order, ...
      |     'arith_type_out', arith_type_out, ...
      |     'bin_pt_out', bin_pt_out);
      settings: AttributesFormatString=|
      | split:[16 16 16 16 16 16 16 16]
      | join:[7 6 5 4 3 2 1 0]
      | Unsigned [128,0]
      mask TypeOptions arith_type_out: Unsigned | Signed  (2's comp) | Floating-point
  munge2 : Subsystem  AncestorBlock=casper_library_flow_control/munge  mask(munge){divisions=8, div_size=[16 16 16 16 16 16 16 16], order=[7 6 5 4 3 2 1 0], arith_type_out=Unsigned, bin_pt_out=0}
      mask prompts: divisions "Number of divisions"; div_size "Division size (bits)"; order "Division packing order"; arith_type_out "Output arithmetic type"; bin_pt_out "Output binary point"
      mask help: Splits an input bus into the specified number of divisions and then recombines them in the order specified (most significant division = 0,least = number divisions-1)
      mask init:
      | munge_init(gcb, ...
      |     'divisions', divisions, ...
      |     'div_size', div_size, ...
      |     'order', order, ...
      |     'arith_type_out', arith_type_out, ...
      |     'bin_pt_out', bin_pt_out);
      settings: AttributesFormatString=|
      | split:[16 16 16 16 16 16 16 16]
      | join:[7 6 5 4 3 2 1 0]
      | Unsigned [128,0]
      mask TypeOptions arith_type_out: Unsigned | Signed  (2's comp) | Floating-point
  munge3 : Subsystem  AncestorBlock=casper_library_flow_control/munge  mask(munge){divisions=8, div_size=[16 16 16 16 16 16 16 16], order=[7 6 5 4 3 2 1 0], arith_type_out=Unsigned, bin_pt_out=0}
      mask prompts: divisions "Number of divisions"; div_size "Division size (bits)"; order "Division packing order"; arith_type_out "Output arithmetic type"; bin_pt_out "Output binary point"
      mask help: Splits an input bus into the specified number of divisions and then recombines them in the order specified (most significant division = 0,least = number divisions-1)
      mask init:
      | munge_init(gcb, ...
      |     'divisions', divisions, ...
      |     'div_size', div_size, ...
      |     'order', order, ...
      |     'arith_type_out', arith_type_out, ...
      |     'bin_pt_out', bin_pt_out);
      settings: AttributesFormatString=|
      | split:[16 16 16 16 16 16 16 16]
      | join:[7 6 5 4 3 2 1 0]
      | Unsigned [128,0]
      mask TypeOptions arith_type_out: Unsigned | Signed  (2's comp) | Floating-point
  munge4 : Subsystem  AncestorBlock=casper_library_flow_control/munge  mask(munge){divisions=8, div_size=[16 16 16 16 16 16 16 16], order=[7 6 5 4 3 2 1 0], arith_type_out=Unsigned, bin_pt_out=0}
      mask prompts: divisions "Number of divisions"; div_size "Division size (bits)"; order "Division packing order"; arith_type_out "Output arithmetic type"; bin_pt_out "Output binary point"
      mask help: Splits an input bus into the specified number of divisions and then recombines them in the order specified (most significant division = 0,least = number divisions-1)
      mask init:
      | munge_init(gcb, ...
      |     'divisions', divisions, ...
      |     'div_size', div_size, ...
      |     'order', order, ...
      |     'arith_type_out', arith_type_out, ...
      |     'bin_pt_out', bin_pt_out);
      settings: AttributesFormatString=|
      | split:[16 16 16 16 16 16 16 16]
      | join:[7 6 5 4 3 2 1 0]
      | Unsigned [128,0]
      mask TypeOptions arith_type_out: Unsigned | Signed  (2's comp) | Floating-point
  munge5 : Subsystem  AncestorBlock=casper_library_flow_control/munge  mask(munge){divisions=8, div_size=[16 16 16 16 16 16 16 16], order=[7 6 5 4 3 2 1 0], arith_type_out=Unsigned, bin_pt_out=0}
      mask prompts: divisions "Number of divisions"; div_size "Division size (bits)"; order "Division packing order"; arith_type_out "Output arithmetic type"; bin_pt_out "Output binary point"
      mask help: Splits an input bus into the specified number of divisions and then recombines them in the order specified (most significant division = 0,least = number divisions-1)
      mask init:
      | munge_init(gcb, ...
      |     'divisions', divisions, ...
      |     'div_size', div_size, ...
      |     'order', order, ...
      |     'arith_type_out', arith_type_out, ...
      |     'bin_pt_out', bin_pt_out);
      settings: AttributesFormatString=|
      | split:[16 16 16 16 16 16 16 16]
      | join:[7 6 5 4 3 2 1 0]
      | Unsigned [128,0]
      mask TypeOptions arith_type_out: Unsigned | Signed  (2's comp) | Floating-point
  munge6 : Subsystem  AncestorBlock=casper_library_flow_control/munge  mask(munge){divisions=8, div_size=[16 16 16 16 16 16 16 16], order=[7 6 5 4 3 2 1 0], arith_type_out=Unsigned, bin_pt_out=0}
      mask prompts: divisions "Number of divisions"; div_size "Division size (bits)"; order "Division packing order"; arith_type_out "Output arithmetic type"; bin_pt_out "Output binary point"
      mask help: Splits an input bus into the specified number of divisions and then recombines them in the order specified (most significant division = 0,least = number divisions-1)
      mask init:
      | munge_init(gcb, ...
      |     'divisions', divisions, ...
      |     'div_size', div_size, ...
      |     'order', order, ...
      |     'arith_type_out', arith_type_out, ...
      |     'bin_pt_out', bin_pt_out);
      settings: AttributesFormatString=|
      | split:[16 16 16 16 16 16 16 16]
      | join:[7 6 5 4 3 2 1 0]
      | Unsigned [128,0]
      mask TypeOptions arith_type_out: Unsigned | Signed  (2's comp) | Floating-point
  munge7 : Subsystem  AncestorBlock=casper_library_flow_control/munge  mask(munge){divisions=8, div_size=[16 16 16 16 16 16 16 16], order=[7 6 5 4 3 2 1 0], arith_type_out=Unsigned, bin_pt_out=0}
      mask prompts: divisions "Number of divisions"; div_size "Division size (bits)"; order "Division packing order"; arith_type_out "Output arithmetic type"; bin_pt_out "Output binary point"
      mask help: Splits an input bus into the specified number of divisions and then recombines them in the order specified (most significant division = 0,least = number divisions-1)
      mask init:
      | munge_init(gcb, ...
      |     'divisions', divisions, ...
      |     'div_size', div_size, ...
      |     'order', order, ...
      |     'arith_type_out', arith_type_out, ...
      |     'bin_pt_out', bin_pt_out);
      settings: AttributesFormatString=|
      | split:[16 16 16 16 16 16 16 16]
      | join:[7 6 5 4 3 2 1 0]
      | Unsigned [128,0]
      mask TypeOptions arith_type_out: Unsigned | Signed  (2's comp) | Floating-point
  munge8 : Subsystem  AncestorBlock=casper_library_flow_control/munge  mask(munge){divisions=8, div_size=[16 16 16 16 16 16 16 16], order=[7 6 5 4 3 2 1 0], arith_type_out=Unsigned, bin_pt_out=0}
      mask prompts: divisions "Number of divisions"; div_size "Division size (bits)"; order "Division packing order"; arith_type_out "Output arithmetic type"; bin_pt_out "Output binary point"
      mask help: Splits an input bus into the specified number of divisions and then recombines them in the order specified (most significant division = 0,least = number divisions-1)
      mask init:
      | munge_init(gcb, ...
      |     'divisions', divisions, ...
      |     'div_size', div_size, ...
      |     'order', order, ...
      |     'arith_type_out', arith_type_out, ...
      |     'bin_pt_out', bin_pt_out);
      settings: AttributesFormatString=|
      | split:[16 16 16 16 16 16 16 16]
      | join:[7 6 5 4 3 2 1 0]
      | Unsigned [128,0]
      mask TypeOptions arith_type_out: Unsigned | Signed  (2's comp) | Floating-point
  munge9 : Subsystem  AncestorBlock=casper_library_flow_control/munge  mask(munge){divisions=8, div_size=[16 16 16 16 16 16 16 16], order=[7 6 5 4 3 2 1 0], arith_type_out=Unsigned, bin_pt_out=0}
      mask prompts: divisions "Number of divisions"; div_size "Division size (bits)"; order "Division packing order"; arith_type_out "Output arithmetic type"; bin_pt_out "Output binary point"
      mask help: Splits an input bus into the specified number of divisions and then recombines them in the order specified (most significant division = 0,least = number divisions-1)
      mask init:
      | munge_init(gcb, ...
      |     'divisions', divisions, ...
      |     'div_size', div_size, ...
      |     'order', order, ...
      |     'arith_type_out', arith_type_out, ...
      |     'bin_pt_out', bin_pt_out);
      settings: AttributesFormatString=|
      | split:[16 16 16 16 16 16 16 16]
      | join:[7 6 5 4 3 2 1 0]
      | Unsigned [128,0]
      mask TypeOptions arith_type_out: Unsigned | Signed  (2's comp) | Floating-point
  offset : Subsystem
  or2 : Subsystem
  packetizer0 : Subsystem  mask{nchan_bits=12, npol_bits=4+1+3, nparallel_bits=6, step_bits=5, time_step_bits=4}
      mask prompts: nchan_bits "Number of channels (including unsent) (2^?)"; npol_bits "Number of pols (2^?)"; nparallel_bits "Parallel samples (2^?)"; step_bits "Step granularity (2^?)"; time_step_bits "Time Steps per cycle (2^?)"
  pfb_ip : xps_library/Utilities/ip  Tag=xps:ip  lib_path=[fileparts(which(bdroot)) '/pfb_fir_4096c_2i_core']  ip_name='pfb_fir_4096c_2i_core'
      settings: SourceProductName=CASPER XPS Blockset
  pipeline0 : Subsystem
  pipeline1 : Subsystem
  pipeline2 : Subsystem
  pipeline3 : Subsystem
  pps_in : xps_library/IO/gpio  Tag=xps:gpio  io_group_params_forwarded=on  io_group=ROACH:led  io_group_real=sync_in  io_group_custom=0  io_dir=in  arith_type=Boolean  bitwidth=1  bin_pt=0  bit_index=0  sample_period=1  use_single_ended=on  use_ddr=off  reg_iob=on  reg_clk_phase=0  termination=None
      settings: SourceProductName=CASPER XPS Blockset
  pulse_ext : Subsystem  AncestorBlock=casper_library_misc/pulse_ext  mask(pulse_ext){pulse_len=2^25}
      mask prompts: pulse_len "Length of Pulse"
      mask help:
      | Extends a boolean signal to be high for the specified number of clocks after
      | the last high input.
      mask init:
      | bits = ceil(log2(pulse_len+1));
      mask Help: eval('xlWeb(''http://casper.berkeley.edu/wiki/Pulse_ext'')')
  pulse_ext1 : Subsystem  AncestorBlock=casper_library_misc/pulse_ext  mask(pulse_ext){pulse_len=2^25}
      mask prompts: pulse_len "Length of Pulse"
      mask help:
      | Extends a boolean signal to be high for the specified number of clocks after
      | the last high input.
      mask init:
      | bits = ceil(log2(pulse_len+1));
      mask Help: eval('xlWeb(''http://casper.berkeley.edu/wiki/Pulse_ext'')')
  reg_in : Subsystem  Tag=xps:sw_reg  AncestorBlock=xps_library/Memory/software_register  mask(swreg){io_dir=From Processor, io_delay=0, init_val=0, sample_period=1, names=reg, bitwidths=32, bin_pts=0, arith_types=0, sim_port=on, show_format=on}
      mask prompts: io_dir "I/O direction"; io_delay "I/O delay"; init_val "Initial Value"; sample_period "Sample period"; names "Bitfield names [msb...lsb]"; bitwidths "Bitfield widths"; bin_pts "Bitfield binary pts"; arith_types "Bitfield types, ufix=0, fix=1, bool=2"; sim_port "Provide sim input/output?"; show_format "Print format string?"
      mask help: A 32-bit software-accessible register. Can be divided into bitfields of varying widths and types using the fields in the block mask.
      mask init:
      | swreg_init(gcb)
      settings: AttributesFormatString=1input:uf32.0 = 32 bits
      mask TypeOptions io_dir: To Processor | From Processor
      mask Callback io_dir:
      | mask_enables = get_param(gcb, 'MaskEnables');
      | mask_names = get_param(gcb, 'MaskNames');
      | if strcmp(get_param(gcb, 'io_dir'), 'To Processor'),
      |     mask_enables{ismember(mask_names, 'sample_period')} = 'off';
      | else
      |     mask_enables{ismember(mask_names, 'sample_period')} = 'on';
      | end
      | set_param(gcb, 'MaskEnables', mask_enables);
      mask DialogControl ParameterTabVar0 Prompt: Setup
  reg_out : Subsystem  Tag=xps:sw_reg  AncestorBlock=xps_library/Memory/software_register  mask(swreg){io_dir=To Processor, io_delay=0, init_val=0, sample_period=1, names=reg, bitwidths=32, bin_pts=0, arith_types=0, sim_port=on, show_format=on}
      mask prompts: io_dir "I/O direction"; io_delay "I/O delay"; init_val "Initial Value"; sample_period "Sample period"; names "Bitfield names [msb...lsb]"; bitwidths "Bitfield widths"; bin_pts "Bitfield binary pts"; arith_types "Bitfield types, ufix=0, fix=1, bool=2"; sim_port "Provide sim input/output?"; show_format "Print format string?"
      mask help: A 32-bit software-accessible register. Can be divided into bitfields of varying widths and types using the fields in the block mask.
      mask init:
      | swreg_init(gcb)
      settings: AttributesFormatString=1output:uf32.0 = 32 bits
      mask TypeOptions io_dir: To Processor | From Processor
      mask Callback io_dir:
      | mask_enables = get_param(gcb, 'MaskEnables');
      | mask_names = get_param(gcb, 'MaskNames');
      | if strcmp(get_param(gcb, 'io_dir'), 'To Processor'),
      |     mask_enables{ismember(mask_names, 'sample_period')} = 'off';
      | else
      |     mask_enables{ismember(mask_names, 'sample_period')} = 'on';
      | end
      | set_param(gcb, 'MaskEnables', mask_enables);
      mask DialogControl ParameterTabVar0 Prompt: Setup
  sel0 : Subsystem  Tag=xps:sw_reg  AncestorBlock=xps_library/Memory/software_register  mask(swreg){io_dir=From Processor, io_delay=0, init_val=0, sample_period=1, names=reg, bitwidths=4, bin_pts=0, arith_types=0, sim_port=on, show_format=on}
      mask prompts: io_dir "I/O direction"; io_delay "I/O delay"; init_val "Initial Value"; sample_period "Sample period"; names "Bitfield names [msb...lsb]"; bitwidths "Bitfield widths"; bin_pts "Bitfield binary pts"; arith_types "Bitfield types, ufix=0, fix=1, bool=2"; sim_port "Provide sim input/output?"; show_format "Print format string?"
      mask help: A 32-bit software-accessible register. Can be divided into bitfields of varying widths and types using the fields in the block mask.
      mask init:
      | swreg_init(gcb)
      settings: AttributesFormatString=1input:uf4.0 = 4 bits
      mask TypeOptions io_dir: To Processor | From Processor
      mask Callback io_dir:
      | mask_enables = get_param(gcb, 'MaskEnables');
      | mask_names = get_param(gcb, 'MaskNames');
      | if strcmp(get_param(gcb, 'io_dir'), 'To Processor'),
      |     mask_enables{ismember(mask_names, 'sample_period')} = 'off';
      | else
      |     mask_enables{ismember(mask_names, 'sample_period')} = 'on';
      | end
      | set_param(gcb, 'MaskEnables', mask_enables);
      mask DialogControl ParameterTabVar0 Prompt: Setup
  sel1 : Subsystem  Tag=xps:sw_reg  AncestorBlock=xps_library/Memory/software_register  mask(swreg){io_dir=From Processor, io_delay=0, init_val=0, sample_period=1, names=reg, bitwidths=4, bin_pts=0, arith_types=0, sim_port=on, show_format=on}
      mask prompts: io_dir "I/O direction"; io_delay "I/O delay"; init_val "Initial Value"; sample_period "Sample period"; names "Bitfield names [msb...lsb]"; bitwidths "Bitfield widths"; bin_pts "Bitfield binary pts"; arith_types "Bitfield types, ufix=0, fix=1, bool=2"; sim_port "Provide sim input/output?"; show_format "Print format string?"
      mask help: A 32-bit software-accessible register. Can be divided into bitfields of varying widths and types using the fields in the block mask.
      mask init:
      | swreg_init(gcb)
      settings: AttributesFormatString=1input:uf4.0 = 4 bits
      mask TypeOptions io_dir: To Processor | From Processor
      mask Callback io_dir:
      | mask_enables = get_param(gcb, 'MaskEnables');
      | mask_names = get_param(gcb, 'MaskNames');
      | if strcmp(get_param(gcb, 'io_dir'), 'To Processor'),
      |     mask_enables{ismember(mask_names, 'sample_period')} = 'off';
      | else
      |     mask_enables{ismember(mask_names, 'sample_period')} = 'on';
      | end
      | set_param(gcb, 'MaskEnables', mask_enables);
      mask DialogControl ParameterTabVar0 Prompt: Setup
  spec_tvg : Subsystem
  ss_adc0 : Subsystem  Tag=casper:snapshot  AncestorBlock=casper_library_scopes/snapshot  mask(snapshot){storage=bram, dram_dimm=1, dram_clock=200, nsamples=10, data_width=128, offset=off, circap=off, value=off, ext_arm=off, ext_circ=off, provide_outputs=on, use_dsp48=off}
      mask prompts: storage "Storage medium"; dram_dimm "DRAM dimm"; dram_clock "DRAM clock rate"; nsamples "Number of Samples (2^?)"; data_width "Data width"; offset "Start delay support"; circap "Circular capture support"; value "Extra value capture support"; ext_arm "External arm support"; ext_circ "External circular capture support"; provide_outputs "Provide outputs"; use_dsp48 "Use DSP48s to implement counters"
      mask help:
      | Standard snap block, but with the following optional extras;
      |  1) Optionally delay the fabric trigger by a user-specified number of valids.
      |  2) Capture continuously after a trigger until a stop pulse is received. Data is captured into BRAM continuously, with old data being overwritten until a stop command is received. Then stop capturing when memory is filled. This enables you to get some data before and some data after the stop pulse. Use the 'tr_en_cnt' register to determine where you are in your vector. 'Addr' register's MSb now indicates 'busy capturing'.
      |  3) Optionally capture a value on an input port to a register at the same time as the first data sample.
      |  4) Implement counters using DSP48Es to save resources.
      mask init:
      | snapshot_init(gcb, ...
      |     'storage', storage, ...
      |     'dram_dimm', dram_dimm, ...
      |     'dram_clock', dram_clock, ...
      |     'nsamples', nsamples, ...
      |     'data_width', data_width, ...
      |     'offset', offset, ...
      |     'circap', circap, ...
      |     'value', value, ...
      |     'ext_arm', ext_arm, ...
      |     'ext_circ', ext_circ, ...
      |     'provide_outputs', 'off', ...
      |     'use_dsp48', use_dsp48);
      settings: AttributesFormatString=|
      | 128 wide, 1024 deep
      | debugID: 76998629
      mask TypeOptions storage: bram | dram
      mask Callback storage: snapshot_callback();
      mask TypeOptions dram_dimm: 1 | 2 | 3 | 4
      mask TypeOptions dram_clock: 200 | 250 | 266 | 300 | 333
      mask TypeOptions data_width: 8 | 16 | 32 | 64 | 128
  ss_adc1 : Subsystem  Tag=casper:snapshot  AncestorBlock=casper_library_scopes/snapshot  mask(snapshot){storage=bram, dram_dimm=1, dram_clock=200, nsamples=10, data_width=128, offset=off, circap=off, value=off, ext_arm=off, ext_circ=off, provide_outputs=on, use_dsp48=off}
      mask prompts: storage "Storage medium"; dram_dimm "DRAM dimm"; dram_clock "DRAM clock rate"; nsamples "Number of Samples (2^?)"; data_width "Data width"; offset "Start delay support"; circap "Circular capture support"; value "Extra value capture support"; ext_arm "External arm support"; ext_circ "External circular capture support"; provide_outputs "Provide outputs"; use_dsp48 "Use DSP48s to implement counters"
      mask help:
      | Standard snap block, but with the following optional extras;
      |  1) Optionally delay the fabric trigger by a user-specified number of valids.
      |  2) Capture continuously after a trigger until a stop pulse is received. Data is captured into BRAM continuously, with old data being overwritten until a stop command is received. Then stop capturing when memory is filled. This enables you to get some data before and some data after the stop pulse. Use the 'tr_en_cnt' register to determine where you are in your vector. 'Addr' register's MSb now indicates 'busy capturing'.
      |  3) Optionally capture a value on an input port to a register at the same time as the first data sample.
      |  4) Implement counters using DSP48Es to save resources.
      mask init: same as zrf_volt_4ant/ss_adc0
      settings: AttributesFormatString=|
      | 128 wide, 1024 deep
      | debugID: 76998629
      mask TypeOptions storage: bram | dram
      mask Callback storage: snapshot_callback();
      mask TypeOptions dram_dimm: 1 | 2 | 3 | 4
      mask TypeOptions dram_clock: 200 | 250 | 266 | 300 | 333
      mask TypeOptions data_width: 8 | 16 | 32 | 64 | 128
  sync : Subsystem
  timebase : Subsystem
  vacc_ss : Subsystem  mask{n_chan_bits=12}
      mask prompts: n_chan_bits "Number of channels (2^?)"
      mask init:
      | ss0 = [gcb '/ss0']
      | ss1 = [gcb '/ss1']
      | 
      | nsamples = num2str(n_chan_bits - 2);
      | 
      | set_param(ss0, 'nsamples', nsamples);
      | set_param(ss1, 'nsamples', nsamples);
  version : Subsystem  Tag=xps:sw_reg  AncestorBlock=xps_library/Memory/software_register  mask(swreg){io_dir=To Processor, io_delay=0, init_val=0, sample_period=1, names=reg, bitwidths=7, bin_pts=0, arith_types=0, sim_port=on, show_format=on}
      mask prompts: io_dir "I/O direction"; io_delay "I/O delay"; init_val "Initial Value"; sample_period "Sample period"; names "Bitfield names [msb...lsb]"; bitwidths "Bitfield widths"; bin_pts "Bitfield binary pts"; arith_types "Bitfield types, ufix=0, fix=1, bool=2"; sim_port "Provide sim input/output?"; show_format "Print format string?"
      mask help: A 32-bit software-accessible register. Can be divided into bitfields of varying widths and types using the fields in the block mask.
      mask init:
      | swreg_init(gcb)
      settings: AttributesFormatString=1output:uf7.0 = 7 bits
      mask TypeOptions io_dir: To Processor | From Processor
      mask Callback io_dir:
      | mask_enables = get_param(gcb, 'MaskEnables');
      | mask_names = get_param(gcb, 'MaskNames');
      | if strcmp(get_param(gcb, 'io_dir'), 'To Processor'),
      |     mask_enables{ismember(mask_names, 'sample_period')} = 'off';
      | else
      |     mask_enables{ismember(mask_names, 'sample_period')} = 'on';
      | end
      | set_param(gcb, 'MaskEnables', mask_enables);
      mask DialogControl ParameterTabVar0 Prompt: Setup
  wires:
  reg_in/1(in_reg) -> Delay/1
  Delay/1 -> reg_out/1(out_reg)
  Constant/1 -> htg_adc_yb/1(m00_axis_tready)
  Constant1/1 -> htg_adc_yb/2(m01_axis_tready)
  Constant2/1 -> htg_adc_yb/3(m02_axis_tready)
  Constant3/1 -> htg_adc_yb/4(m03_axis_tready)
  Constant4/1 -> htg_adc_yb/5(m10_axis_tready)
  Constant5/1 -> htg_adc_yb/6(m11_axis_tready)
  Constant6/1 -> htg_adc_yb/7(m12_axis_tready)
  Constant7/1 -> htg_adc_yb/8(m13_axis_tready)
  Constant8/1 -> htg_adc_yb/9(m20_axis_tready)
  Constant9/1 -> htg_adc_yb/10(m21_axis_tready)
  Constant10/1 -> htg_adc_yb/11(m22_axis_tready)
  Constant11/1 -> htg_adc_yb/12(m23_axis_tready)
  Constant14/1 -> htg_adc_yb/13(m30_axis_tready)
  Constant15/1 -> htg_adc_yb/14(m31_axis_tready)
  Constant12/1 -> htg_adc_yb/15(m32_axis_tready)
  Constant13/1 -> htg_adc_yb/16(m33_axis_tready)
  Constant17/1 -> deadbeef/1(out_reg)
  count_rst/1(in_reg) -> Counter2/1
  Counter2/1 -> Delay3/1
  Delay3/1 -> count_out/1(out_reg)
  adc_rstn/1(in_reg) -> htg_adc_yb/17(rstn)
  [x0] -> ss_adc0/1(din)
  Constant19/1 -> [adc_sync_out]
  Constant18/1 -> ss_adc0/3(trig)
  Delay18/1 -> [x0]
  Constant16/1 -> ss_adc0/2(we)
  Constant20/1 -> ss_adc1/2(we)
  Constant21/1 -> ss_adc1/3(trig)
  [y0] -> ss_adc1/1(din)
  pulse_ext1/1(out) -> led1/1
  sync/1(sync_gpio_in) -> timebase/1(sync_gpio_in)
  sync/3(arm_sync) -> timebase/3(arm_sync)
  [mrst] -> led2/1
  [sync_gen] -> pulse_ext1/1(in)
  [sync_trig] -> pulse_ext/1(in)
  Constant22/1 -> Slice2/1, version/1(out_reg)
  timebase/1(sync_in) -> [sync_trig]
  Slice2/1 -> [version]
  timebase/3(mrst) -> [mrst]
  [adc_sync_out] -> sync/1(ext_sync0)
  pulse_ext/1(out) -> led0/1
  sync/2(sw_sync) -> timebase/2(sw_sync)
  timebase/2(sync_gen) -> [sync_gen]
  Delay21/1 -> eth0/2(vld)
  Delay23/1 -> eth0/4(dest_ip)
  Delay20/1 -> eth0/1(data)
  Delay22/1 -> eth0/3(eof)
  htg_adc_yb/1(m00_axis_tdata) -> munge2/1(din)
  htg_adc_yb/3(m01_axis_tdata) -> munge3/1(din)
  htg_adc_yb/5(m02_axis_tdata) -> munge4/1(din)
  htg_adc_yb/7(m03_axis_tdata) -> munge5/1(din)
  htg_adc_yb/9(m10_axis_tdata) -> munge6/1(din)
  htg_adc_yb/11(m11_axis_tdata) -> munge7/1(din)
  htg_adc_yb/13(m12_axis_tdata) -> munge8/1(din)
  htg_adc_yb/15(m13_axis_tdata) -> munge9/1(din)
  htg_adc_yb/17(m20_axis_tdata) -> munge10/1(din)
  htg_adc_yb/19(m21_axis_tdata) -> munge11/1(din)
  htg_adc_yb/21(m22_axis_tdata) -> munge12/1(din)
  htg_adc_yb/23(m23_axis_tdata) -> munge13/1(din)
  htg_adc_yb/25(m30_axis_tdata) -> munge14/1(din)
  htg_adc_yb/27(m31_axis_tdata) -> munge15/1(din)
  htg_adc_yb/29(m32_axis_tdata) -> munge16/1(din)
  htg_adc_yb/31(m33_axis_tdata) -> munge17/1(din)
  htg_adc_yb/2(m00_axis_tvalid) -> [in8_vld]
  htg_adc_yb/4(m01_axis_tvalid) -> [in16_vld]
  htg_adc_yb/6(m02_axis_tvalid) -> [in7_vld]
  htg_adc_yb/8(m03_axis_tvalid) -> [in15_vld]
  htg_adc_yb/10(m10_axis_tvalid) -> [in6_vld]
  htg_adc_yb/12(m11_axis_tvalid) -> [in14_vld]
  htg_adc_yb/14(m12_axis_tvalid) -> [in5_vld]
  htg_adc_yb/16(m13_axis_tvalid) -> [in13_vld]
  htg_adc_yb/18(m20_axis_tvalid) -> [in4_vld]
  htg_adc_yb/20(m21_axis_tvalid) -> [in12_vld]
  htg_adc_yb/22(m22_axis_tvalid) -> [in3_vld]
  htg_adc_yb/24(m23_axis_tvalid) -> [in11_vld]
  htg_adc_yb/26(m30_axis_tvalid) -> [in2_vld]
  htg_adc_yb/28(m31_axis_tvalid) -> [in10_vld]
  htg_adc_yb/30(m32_axis_tvalid) -> [in1_vld]
  htg_adc_yb/32(m33_axis_tvalid) -> [in9_vld]
  sel0/1(in_reg) -> Delay1/1
  Delay1/1 -> Mux/1
  [in1] -> Mux/2
  [in2] -> Mux/3
  [in3] -> Mux/4
  [in4] -> Mux/5
  [in5] -> Mux/6
  [in6] -> Mux/7
  [in7] -> Mux/8
  [in8] -> Mux/9
  [in9] -> Mux/10
  [in10] -> Mux/11
  [in11] -> Mux/12
  [in12] -> Mux/13
  [in13] -> Mux/14
  [in14] -> Mux/15
  [in15] -> Mux/16
  [in16] -> Mux/17
  [in16] -> Mux1/17
  [in15] -> Mux1/16
  [in14] -> Mux1/15
  [in13] -> Mux1/14
  [in12] -> Mux1/13
  [in11] -> Mux1/12
  [in10] -> Mux1/11
  [in9] -> Mux1/10
  [in8] -> Mux1/9
  [in7] -> Mux1/8
  [in6] -> Mux1/7
  [in5] -> Mux1/6
  [in4] -> Mux1/5
  [in3] -> Mux1/4
  [in2] -> Mux1/3
  [in1] -> Mux1/2
  Delay2/1 -> Mux1/1
  sel1/1(in_reg) -> Delay2/1
  Delay4/1 -> [y0]
  Mux/1 -> Delay18/1
  Mux1/1 -> Delay4/1
  munge2/1(dout) -> [in8]
  munge3/1(dout) -> [in16]
  munge4/1(dout) -> [in7]
  munge5/1(dout) -> [in15]
  munge6/1(dout) -> [in6]
  munge7/1(dout) -> [in14]
  munge8/1(dout) -> [in5]
  munge9/1(dout) -> [in13]
  munge10/1(dout) -> [in4]
  munge11/1(dout) -> [in12]
  munge12/1(dout) -> [in3]
  munge13/1(dout) -> [in11]
  munge14/1(dout) -> [in2]
  munge15/1(dout) -> [in10]
  munge16/1(dout) -> [in1]
  munge17/1(dout) -> [in9]
  [sync_gen] -> pipeline0/1(sync_in)
  [mrst] -> pipeline0/4(mrst)
  [version] -> pipeline0/5(version)
  Delay5/1 -> eth0/6(byte_enable)
  [in1] -> pipeline0/2(x)
  [in2] -> pipeline0/3(y)
  pps_in/1 -> edge_detect/1(in)
  [in4] -> pipeline1/3(y)
  [in3] -> pipeline1/2(x)
  [version] -> pipeline1/5(version)
  [mrst] -> pipeline1/4(mrst)
  [sync_gen] -> pipeline1/1(sync_in)
  [sync_gen] -> pipeline2/1(sync_in)
  [mrst] -> pipeline2/4(mrst)
  [version] -> pipeline2/5(version)
  [in5] -> pipeline2/2(x)
  [in6] -> pipeline2/3(y)
  [in7] -> pipeline3/2(x)
  [in8] -> pipeline3/3(y)
  [sync_gen] -> pipeline3/1(sync_in)
  [mrst] -> pipeline3/4(mrst)
  [version] -> pipeline3/5(version)
  byte_flip/1(dout) -> Delay20/1
  Delay7/1 -> eth0/5(dest_port)
  edge_detect/1(out) -> sync/2(ext_sync1)
  corr/1(ss_vld_out) -> vacc_ss/1(vld)
  corr/2(ss_dout) -> vacc_ss/2(xx_yy_xy)
  spec_tvg/2(dout) -> corr/2(din)
  spec_tvg/1(sync_out) -> corr/1(sync)
  [mrst] -> packetizer0/3(mrst_in)
  chan_reorder/2(dout0) -> offset/1(din)
  offset/1(dout) -> packetizer0/2(data_in)
  Constant23/1 -> Concat1/1
  [version] -> Concat1/2
  Concat1/1 -> packetizer0/4(version)
  chan_reorder/1(sync_out) -> packetizer0/1(sync_in)
  or2/1(Out1) -> spec_tvg/2(din)
  pipeline0/3(pfb_sync_out) -> [pfb_sync_out]
  [pfb_sync_out] -> Delay6/1
  Delay6/1 -> spec_tvg/1(sync)
  pipeline0/4(pfb_dout) -> [pfb_dout0]
  pipeline1/4(pfb_dout) -> [pfb_dout1]
  pipeline2/4(pfb_dout) -> [pfb_dout2]
  pipeline3/4(pfb_dout) -> [pfb_dout3]
  [pfb_dout0] -> or2/1(In1)
  [pfb_dout2] -> or2/7(In7)
  [pfb_dout1] -> or2/6(In6)
  [pfb_dout0] -> or2/5(In5)
  [pfb_dout1] -> or2/2(In2)
  [pfb_dout2] -> or2/3(In3)
  [pfb_dout3] -> or2/4(In4)
  [pfb_dout3] -> or2/8(In8)
  [mrst] -> corr/3(mrst)
  packetizer0/1(data_out) -> byte_flip/1(din)
  packetizer0/2(valid_out) -> Delay21/1
  packetizer0/3(eof) -> Delay22/1
  packetizer0/4(dest_ip) -> Delay23/1
  packetizer0/5(dest_port) -> Delay7/1
  packetizer0/6(byte_enable) -> Delay5/1
  pipeline0/1(sync_out) -> [sync0]
  [sync0] -> chan_reorder/1(sync)
  pipeline0/2(dout) -> [dout0]
  pipeline1/2(dout) -> [dout1]
  pipeline2/2(dout) -> [dout2]
  pipeline3/2(dout) -> [dout3]
  [dout0] -> chan_reorder/3(din0)
  [dout1] -> chan_reorder/4(din1)
  [mrst] -> chan_reorder/2(mrst)
  [dout2] -> chan_reorder/5(din2)
  [dout3] -> chan_reorder/6(din3)
  dup2/1(Out1) -> chan_reorder/7(din4)
  dup3/1(Out1) -> chan_reorder/8(din5)
  dup4/1(Out1) -> chan_reorder/9(din6)
  dup5/1(Out1) -> chan_reorder/10(din7)
  Constant26/1 -> dup2/1(In1)
  Constant29/1 -> dup5/1(In1)
  Constant27/1 -> dup3/1(In1)
  Constant28/1 -> dup4/1(In1)
